simulink model "simulink_b3"  (R2022b)
settings: Solver=VariableStepAuto  StartTime=0.0  StopTime=2  RelTol=1e-3
PreLoadFcn:
  | progetto.m
model workspace: external: MAT-File /Users/alberto/Documents/MATLAB/CAT/progetto.mat (data not in the file)
values from neighbouring files (symbols this model uses):
  alfa = 0.5    [GraficoAnimato.m]    (also in progetto.m)
  beta = 0.8    [GraficoAnimato.m]    (also in progetto.m)
  gamma = 0.2    [GraficoAnimato.m]    (also in progetto.m)
  K = 500    [GraficoAnimato.m]    (also in progetto.m)
  mr = 0.05    [GraficoAnimato.m]    (also in progetto.m)
  ms = 0.95    [GraficoAnimato.m]    (also in progetto.m)
  rr = 1.4    [GraficoAnimato.m]    (also in progetto.m)
  rs = 1.7    [GraficoAnimato.m]    (also in progetto.m)
  x1_e = 100    [progetto.m]
  x2_e = 400    [progetto.m]
libraries: cstblocks x2
settings Model: Creator=alberto  LastModifiedBy=alberto
settings SolverCC: MaxConsecutiveMinStep=2

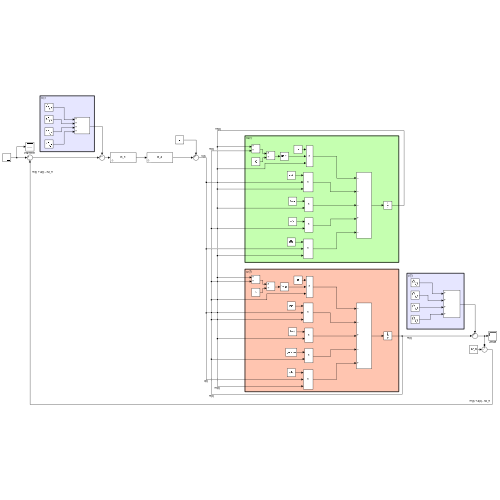
[thumbnail: Simulink's stored preview of the top-level diagram]
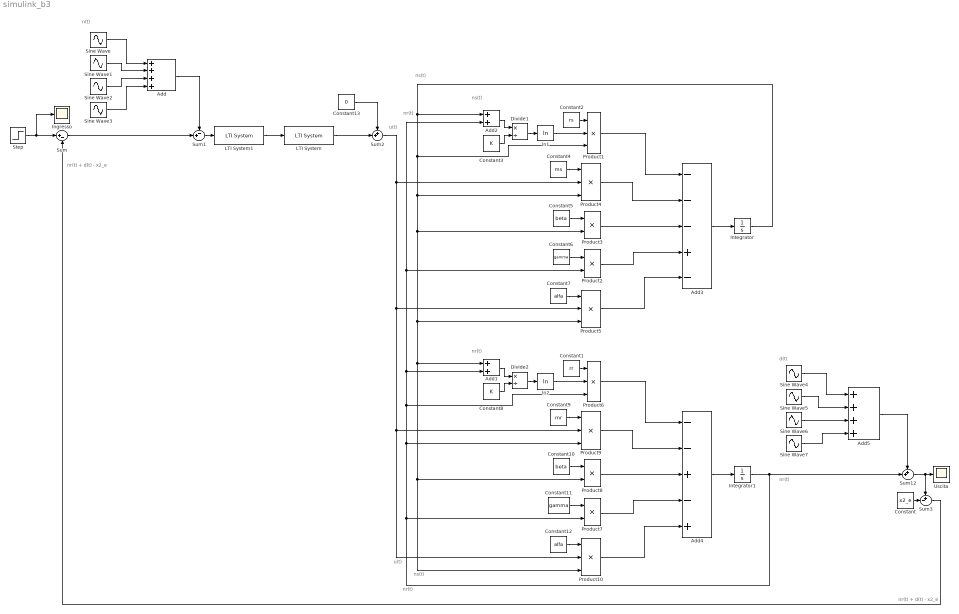
== system simulink_b3 ==
  note: nr(t)
  note: ns(t)
  note: nr(t)
  note: u(t)
  note: nr(t)
  note: ns(t)
  note: u(t)
  note: ns(t)
  note: d(t)
  note: n(t)
  note: nr(t)
  note: nr(t) + d(t) - x2_e
  note: nr(t) + d(t) - x2_e
  Add : Sum  Inputs=++++
  Add1 : Sum
  Add2 : Sum
  Add3 : Sum  Inputs=---+-
  Add4 : Sum  Inputs=--+-+
  Add5 : Sum  Inputs=++++
  Constant : Constant  Value=x2_e
  Constant1 : Constant  Value=rr
  Constant10 : Constant  Value=beta
  Constant11 : Constant  Value=gamma
  Constant12 : Constant  Value=alfa
  Constant13 : Constant  Value=0
  Constant2 : Constant  Value=rs
  Constant3 : Constant  Value=K
  Constant4 : Constant  Value=ms
  Constant5 : Constant  Value=beta
  Constant6 : Constant  Value=gamma
  Constant7 : Constant  Value=alfa
  Constant8 : Constant  Value=K
  Constant9 : Constant  Value=mr
  Divide1 : Product  Inputs=*/
  Divide2 : Product  Inputs=*/
  Ingresso : Scope
      settings: Tag=Ingresso
  Integrator : Integrator  InitialCondition=x1_e
  Integrator1 : Integrator  InitialCondition=x2_e
  LTI System : cstblocks/LTI System  sys=R_d  IC=[]
  LTI System1 : cstblocks/LTI System  sys=R_s  IC=[]
  Product{1,4..6,9..10} (6 alike) : Product  Inputs=3
  Product{2..3,7..8} (4 alike) : Product
  Sine Wave : Sin  Amplitude=0.1  Frequency=(5*10^3)*1  SampleTime=0
  Sine Wave1 : Sin  Amplitude=0.1  Frequency=(5*10^3)*2  SampleTime=0
  Sine Wave2 : Sin  Amplitude=0.1  Frequency=(5*10^3)*3  SampleTime=0
  Sine Wave3 : Sin  Amplitude=0.1  Frequency=(5*10^3)*4  SampleTime=0
  Sine Wave4 : Sin  Amplitude=0.2  Frequency=0.025*1  SampleTime=0
  Sine Wave5 : Sin  Amplitude=0.2  Frequency=0.025*2  SampleTime=0
  Sine Wave6 : Sin  Amplitude=0.2  Frequency=0.025*3  SampleTime=0
  Sine Wave7 : Sin  Amplitude=0.2  Frequency=0.025*4  SampleTime=0
  Step : Step  Time=0  After=-3  SampleTime=0
  Sum : Sum  Inputs=|+-
  Sum1 : Sum  Inputs=-+|
  Sum12 : Sum  Inputs=++|
  Sum2 : Sum  Inputs=++|
  Sum3 : Sum  Inputs=+-|
  Uscita : Scope
      settings: Tag=Uscita
  ln1 : Math  Operator=log
  ln2 : Math  Operator=log
  wires:
  Sum/1 -> Sum1/2
  Sum1/1 -> LTI System1/1
  Sine Wave/1 -> Add/1
  Sine Wave1/1 -> Add/2
  Sine Wave2/1 -> Add/3
  Sine Wave3/1 -> Add/4
  Sine Wave7/1 -> Add5/4
  Sine Wave4/1 -> Add5/1
  Sine Wave5/1 -> Add5/2
  Sine Wave6/1 -> Add5/3
  Sum12/1 -> Sum3/1, Uscita/1
  Divide1/1 -> ln1/1
  Add2/1 -> Divide1/1
  Constant3/1 -> Divide1/2
  Constant2/1 -> Product1/1
  ln1/1 -> Product1/2
  Constant5/1 -> Product3/1
  Constant4/1 -> Product4/1
  Constant6/1 -> Product2/1
  Constant7/1 -> Product5/1
  Product1/1 -> Add3/1
  Product4/1 -> Add3/2
  Product3/1 -> Add3/3
  Product2/1 -> Add3/4
  Product5/1 -> Add3/5
  Constant9/1 -> Product9/1
  Constant11/1 -> Product7/1
  Divide2/1 -> ln2/1
  Constant1/1 -> Product6/1
  Product7/1 -> Add4/4
  Product6/1 -> Add4/1
  Product10/1 -> Add4/5
  Product9/1 -> Add4/2
  Constant10/1 -> Product8/1
  Product8/1 -> Add4/3
  Constant8/1 -> Divide2/2
  ln2/1 -> Product6/2
  Add1/1 -> Divide2/1
  Constant12/1 -> Product10/1
  Add4/1 -> Integrator1/1
  Add3/1 -> Integrator/1
  Integrator1/1 -> Sum12/2, Product7/2, Product9/3, Product6/3, Add1/2, Product2/2, Add2/2
  Integrator/1 -> Add1/1, Product10/3, Product8/2, Product5/3, Product3/2, Product4/3, Product1/3, Add2/1
  LTI System/1 -> Sum2/2
  Sum2/1 -> Product10/2, Product9/2, Product5/2, Product4/2
  Constant13/1 -> Sum2/1
  Constant/1 -> Sum3/2
  Sum3/1 -> Sum/2
  LTI System1/1 -> LTI System/1
  Add/1 -> Sum1/1
  Add5/1 -> Sum12/1
  Step/1 -> Ingresso/1, Sum/1
